simulink model "B_SIMU_LazoCerrado_PI"  (R2017a)
settings: Solver=VariableStepAuto  StartTime=0.0  StopTime=1500  RelTol=1e-3
libraries: simulink x1
settings Model: Creator=pablo  LastModifiedBy=pablo

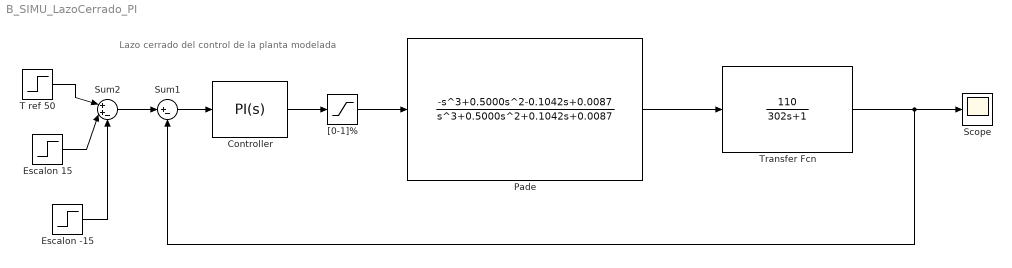
== system B_SIMU_LazoCerrado_PI ==
  note: Lazo cerrado del control de la planta modelada
  " Controller" : simulink/Continuous/PID Controller  Controller=PI  TimeDomain=Continuous-time  SampleTime=-1  IntegratorMethod=Forward Euler  FilterMethod=Forward Euler  Form=Parallel  UseFilter=on  ControllerParametersSource=internal  P=0.1  I=0.0001  D=0  N=100  InitialConditionSource=internal  InitialConditionForIntegrator=0  InitialConditionForFilter=0  ExternalReset=none  LimitOutput=on  UpperSaturationLimit=inf  LowerSaturationLimit=0  LinearizeAsGain=on  AntiWindupMode=none  Kb=1  TrackingMode=off  Kt=1  PParamMin=[]  PParamMax=[]  IParamMin=[]  IParamMax=[]  DParamMin=[]  DParamMax=[]  NParamMin=[]  NParamMax=[]  KbParamMin=[]  KbParamMax=[]  KtParamMin=[]  KtParamMax=[]  POutMin=[]  POutMax=[]  IOutMin=[]  IOutMax=[]  DOutMin=[]  DOutMax=[]  NOutMin=[]  NOutMax=[]  KbOutMin=[]  KbOutMax=[]  KtOutMin=[]  KtOutMax=[]  IntegratorOutMin=[]  IntegratorOutMax=[]  FilterOutMin=[]  FilterOutMax=[]  SumOutMin=[]  SumOutMax=[]  SumI1OutMin=[]  SumI1OutMax=[]  SumI2OutMin=[]  SumI2OutMax=[]  SumI3OutMin=[]  SumI3OutMax=[]  SumDOutMin=[]  SumDOutMax=[]  SaturationOutMin=[]  SaturationOutMax=[]  IntegratorContinuousStateAttributes=''  IntegratorStateMustResolveToSignalObject=off  IntegratorRTWStateStorageClass=Auto  FilterContinuousStateAttributes=''  FilterStateMustResolveToSignalObject=off  FilterRTWStateStorageClass=Auto  DifferentiatorICPrevScaledInput=0  DifferentiatorOutMin=[]  DifferentiatorOutMax=[]  InitialConditionSetting=State (most efficient)
  Escalon -15 : Step  Time=1000  After=15  SampleTime=0
  Escalon 15 : Step  Time=500  After=15  SampleTime=0
  Pade : TransferFcn  Numerator="[-1.0000    0.5000    -0.1042    0.0087]"  Denominator="[1.0000    0.5000    0.1042    0.0087]"
  Scope : Scope
  Sum1 : Sum  Inputs=|+-
  Sum2 : Sum  Inputs=|++-
  T ref 50 : Step  Time=0  After=50  SampleTime=0
  Transfer Fcn : TransferFcn  Numerator=[110]  Denominator=[302 1]
  "[0-1]%" : Saturate  UpperLimit=1  LowerLimit=0
  wires:
  Pade/1 -> Transfer Fcn/1
  Transfer Fcn/1 -> Sum1/2, Scope/1
  " Controller"/1 -> "[0-1]%"/1
  "[0-1]%"/1 -> Pade/1
  T ref 50/1 -> Sum2/1
  Escalon 15/1 -> Sum2/2
  Sum1/1 -> " Controller"/1
  Sum2/1 -> Sum1/1
  Escalon -15/1 -> Sum2/3
